simulink model "TRN_visualization"  (R2020b)
settings: Solver=FixedStepDiscrete  StartTime=0.0  StopTime=10.0  FixedStep=0.04  RelTol=1e-3
libraries: simulink_extras x3
settings Model: Creator=wnstj  LastModifiedBy=ASCL
settings OptimizationCC: DefaultParameterBehavior=Inlined  UseDivisionForNetSlopeComputation=on  GainParamInheritBuiltInType=on  UseFloatMulNetSlope=on  InlineInvariantSignals=on  PassReuseOutputArgsAs=Individual arguments  ZeroExternalMemoryAtStartup=off  ZeroInternalMemoryAtStartup=off  NoFixptDivByZeroProtection=on  EfficientFloat2IntCast=on  LifeSpan=1  OptimizeBlockOrder=speed  DifferentSizesBufferReuse=on  EfficientTunableParamExpr=on
settings DebuggingCC: ParameterTunabilityLossMsg=error  SFUnexpectedBacktrackingDiag=warning  SFNoUnconditionalDefaultTransitionDiag=warning  SFMachineParentedDataDiag=error
settings HardwareCC: ProdBitPerPointer=32  ProdBitPerSizeT=32  ProdBitPerPtrDiffT=32  ProdLargestAtomicInteger=Long  ProdLargestAtomicFloat=Double  ProdEndianess=BigEndian  ProdWordSize=32  ProdLongLongMode=on  ProdHWDeviceType=Freescale->MPC83xx
settings ModelReferenceCC: ModelReferenceNumInstancesAllowed=Single
settings SFSimCC: MATLABDynamicMemAlloc=off
settings RTWCC: Description=Embedded Coder  SystemTargetFile=ert.tlc  TemplateMakefile=ert_default_tmf  BuildConfiguration=Debug
settings CodeAppCC: ForceParamTrailComments=on  IgnoreCustomStorageClasses=off  OperatorAnnotations=on  SimulinkDataObjDesc=on  SFDataObjDesc=on  InsertBlockDesc=on
settings ERTTargetCC: TargetLangStandard=C99 (ISO)  GenerateSampleERTMain=on  IncludeMdlTerminateFcn=off  CombineSignalStateStructs=on  SupportAbsoluteTime=off  SupportComplex=off  InlinedParameterPlacement=NonHierarchical  ERTCustomFileTemplate=example_file_process.tlc  ERTFilePackagingFormat=CompactWithDataFile

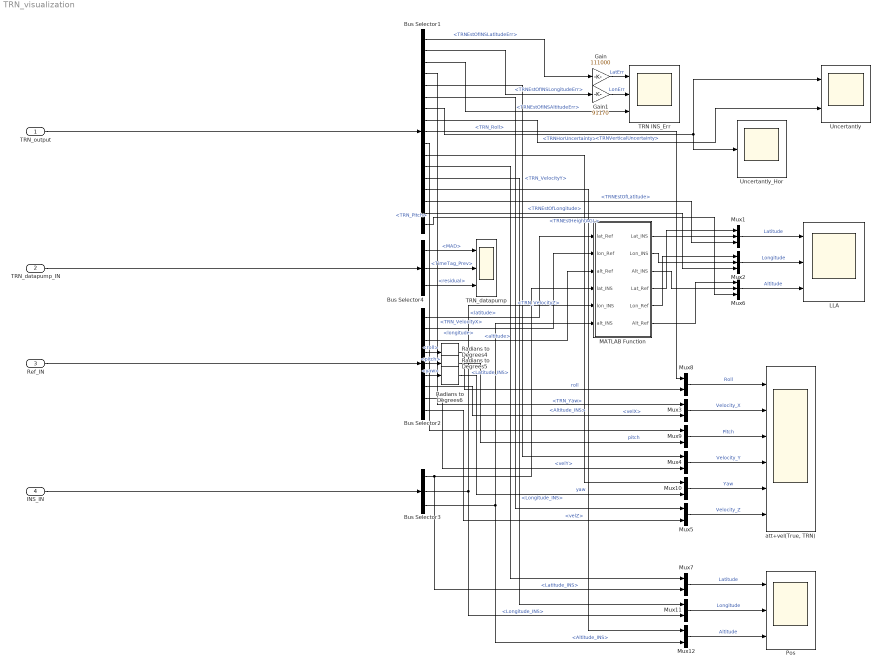
== system TRN_visualization ==
  TRN_output : Inport  OutDataTypeStr=Bus: TRNOutput
  TRN_datapump_IN : Inport  Port=2  OutDataTypeStr=Bus: TRNDatapump
  Ref_IN : Inport  Port=3  OutDataTypeStr=Bus: BUS_DYN_STATE
  INS_IN : Inport  Port=4  OutDataTypeStr=Bus: TRNInput
  Bus Selector1 : BusSelector  OutputSignals=TRNEstOfINSLatitudeErr,TRNEstOfINSLongitudeErr,TRNEstOfINSAltitudeErr,TRN_VelocityX,TRN_VelocityY,TRN_VelocityZ,TRNHorUncertainty,TRNVerticalUncertainty,TRN_Roll,TRN_Pitch,TRN_Yaw,Latitude_INS,Longitude_INS,Altitude_INS,TRNEstOfLatitude,TRNEstOfLongitude,TRNEstHeightAGL
  Bus Selector2 : BusSelector  OutputSignals=latitude,longitude,altitude,roll,pitch,yaw,velX,velY,velZ
  Bus Selector3 : BusSelector  OutputSignals=Latitude_INS,Longitude_INS,Altitude_INS
  Bus Selector4 : BusSelector  OutputSignals=MAD,TimeTag_Prev,residual
  Gain : Gain  Gain=111000
  Gain1 : Gain  Gain=91170
  LLA : Scope  NumInputPorts=3
  MATLAB Function : MATLAB Function  TreatAsAtomicUnit=on
  Mux1 : Mux  Inputs=3
  Mux{3..5,7..12} (9 alike) : Mux  Inputs=2
  Mux2 : Mux  Inputs=3
  Mux6 : Mux  Inputs=3
  Pos : Scope  NumInputPorts=3
  Radians to Degrees4 : simulink_extras/Transformations/Radians to Degrees
  Radians to Degrees5 : simulink_extras/Transformations/Radians to Degrees
  Radians to Degrees6 : simulink_extras/Transformations/Radians to Degrees
  TRN INS_Err : Scope  NumInputPorts=3
  TRN_datapump : Scope  NumInputPorts=3
  Uncertantly : Scope  NumInputPorts=2
  Uncertantly_Hor : Scope
  "att+vel(True, TRN)" : Scope  NumInputPorts=6
  wires:
  Bus Selector3/1 -> MATLAB Function/4(lat_INS), Mux7/2  "<Latitude_INS>"
  Bus Selector3/2 -> MATLAB Function/5(lon_INS), Mux11/2  "<Longitude_INS>"
  Bus Selector4/3 -> TRN_datapump/3  "<residual>"
  TRN_output/1 -> Bus Selector1/1
  Bus Selector4/1 -> TRN_datapump/1  "<MAD>"
  Bus Selector1/4 -> Mux3/1  "<TRN_VelocityX>"
  Bus Selector1/7 -> Uncertantly/1, Uncertantly_Hor/1  "<TRNHorUncertainty>"
  Gain/1 -> TRN INS_Err/1  "LatErr"
  Bus Selector4/2 -> TRN_datapump/2  "<TimeTag_Prev>"
  Bus Selector1/1 -> Gain/1  "<TRNEstOfINSLatitudeErr>"
  MATLAB Function/6(Alt_Ref) -> Mux6/1
  Bus Selector2/3 -> MATLAB Function/3(alt_Ref)  "<altitude>"
  Mux2/1 -> LLA/2  "Longitude"
  Mux1/1 -> LLA/1  "Latitude"
  Bus Selector2/2 -> MATLAB Function/2(lon_Ref)  "<longitude>"
  Bus Selector2/1 -> MATLAB Function/1(lat_Ref)  "<latitude>"
  Bus Selector3/3 -> Mux12/2, MATLAB Function/6(alt_INS)  "<Altitude_INS>"
  Ref_IN/1 -> Bus Selector2/1
  Gain1/1 -> TRN INS_Err/2  "LonErr"
  Bus Selector1/3 -> TRN INS_Err/3  "<TRNEstOfINSAltitudeErr>"
  Bus Selector1/6 -> Mux5/1  "<TRN_VelocityZ>"
  Bus Selector1/5 -> Mux4/1  "<TRN_VelocityY>"
  Bus Selector1/2 -> Gain1/1  "<TRNEstOfINSLongitudeErr>"
  TRN_datapump_IN/1 -> Bus Selector4/1
  INS_IN/1 -> Bus Selector3/1
  MATLAB Function/1(Lat_INS) -> Mux1/2
  MATLAB Function/2(Lon_INS) -> Mux2/2
  MATLAB Function/3(Alt_INS) -> Mux6/2
  Mux3/1 -> "att+vel(True, TRN)"/2  "Velocity_X"
  Mux4/1 -> "att+vel(True, TRN)"/4  "Velocity_Y"
  Mux5/1 -> "att+vel(True, TRN)"/6  "Velocity_Z"
  Bus Selector2/7 -> Mux3/2  "<velX>"
  Bus Selector2/8 -> Mux4/2  "<velY>"
  Bus Selector2/9 -> Mux5/2  "<velZ>"
  Mux8/1 -> "att+vel(True, TRN)"/1  "Roll"
  Bus Selector1/9 -> Mux8/1  "<TRN_Roll>"
  Mux9/1 -> "att+vel(True, TRN)"/3  "Pitch"
  Bus Selector1/10 -> Mux9/1  "<TRN_Pitch>"
  Bus Selector1/11 -> Mux10/1  "<TRN_Yaw>"
  Mux10/1 -> "att+vel(True, TRN)"/5  "Yaw"
  Radians to Degrees6/1 -> Mux10/2  "yaw"
  Radians to Degrees4/1 -> Mux8/2  "roll"
  Radians to Degrees5/1 -> Mux9/2  "pitch"
  Bus Selector2/4 -> Radians to Degrees4/1  "<roll>"
  Bus Selector2/5 -> Radians to Degrees5/1  "<pitch>"
  Bus Selector2/6 -> Radians to Degrees6/1  "<yaw>"
  Mux7/1 -> Pos/1  "Latitude"
  Mux11/1 -> Pos/2  "Longitude"
  Mux12/1 -> Pos/3  "Altitude"
  Bus Selector1/12 -> Mux7/1  "<Latitude_INS>"
  Bus Selector1/13 -> Mux11/1  "<Longitude_INS>"
  Bus Selector1/14 -> Mux12/1  "<Altitude_INS>"
  MATLAB Function/5(Lon_Ref) -> Mux2/1
  MATLAB Function/4(Lat_Ref) -> Mux1/1
  Bus Selector1/8 -> Uncertantly/2  "<TRNVerticalUncertainty>"
  Mux6/1 -> LLA/3  "Altitude"
  Bus Selector1/15 -> Mux1/3  "<TRNEstOfLatitude>"
  Bus Selector1/16 -> Mux2/3  "<TRNEstOfLongitude>"
  Bus Selector1/17 -> Mux6/3  "<TRNEstHeightAGL>"

== matlab function TRN_visualization/MATLAB Function ==
  data: lat_Ref input; lon_Ref input; alt_Ref input; lat_INS input; lon_INS input; alt_INS input; Lat_INS output; Lon_INS output; Alt_INS output; Lat_Ref output; Lon_Ref output; Alt_Ref output
function [Lat_INS, Lon_INS, Alt_INS, Lat_Ref, Lon_Ref, Alt_Ref] = fcn(lat_Ref, lon_Ref, alt_Ref, lat_INS, lon_INS, alt_INS)

%% parameters
% lat2m = 111000;
% lon2m = 91170;

%% 초기값 setting
% init_lat = 35.1;
% init_lon = 128.5;
% init_alt = 1000;

Lat_INS = lat_INS;               % INS Latitude
Lon_INS = lon_INS;               % INS Longitude
Alt_INS = uint16(alt_INS);               % INS Altitude

Lat_Ref = lat_Ref;             % Ref Latitude
Lon_Ref = lon_Ref;             % Ref Longitude
Alt_Ref = uint16(alt_Ref);             % Ref Altitude


end
